simulink model "Fishhook"  (R2018a)
settings: Solver=FixedStepDiscrete  StartTime=0.0  StopTime=1  FixedStep=0.001  RelTol=1e-3  EnableMultiTasking=on
values from neighbouring files (symbols this model uses):
  DLCTest = [0 0 0 0 0 0 0 0 0 0 0 0 ... (12003 elements, 12003x1)]    [DLCTest.mat]
  Ts = 0.001    [ISData.m]    (also in IS_2impulse.m; IS_3impulse.m; IS_4impulse.m; InputShaper.m)
undefined symbols (not defined in the file or in its folder): theta_sw_FH
settings Model: ExtModeTrigDuration=10000  Creator=srivats  LastModifiedBy=srivats
settings SolverCC: PositivePriorityOrder=on
settings RTWCC: SystemTargetFile=quarc_win64.tlc  TemplateMakefile=quarc_default_tmf  Description=QUARC Win64 Target
settings STFCustomTargetCC: TargetPreCompLibLocation=C:\PROGRA~3\QUARC\lib\2018a\win64\release  TargetLangStandard=C99 (ISO)  ConcurrentExecutionCompliant=on  SystemTargetFile=quarc_win64.tlc
settings GRTTargetCC: TargetPreCompLibLocation=C:\PROGRA~3\QUARC\lib\2018a\win64\release  ParMdlRefBuildCompliant=off  CompOptLevelCompliant=off  CombineOutputUpdateFcns=off  MatFileLogging=off  CPPClassGenCompliant=off  GRTInterface=on  UseToolchainInfoCompliant=off  ExtMode=on  ExtModeMexFile=quarc_comm

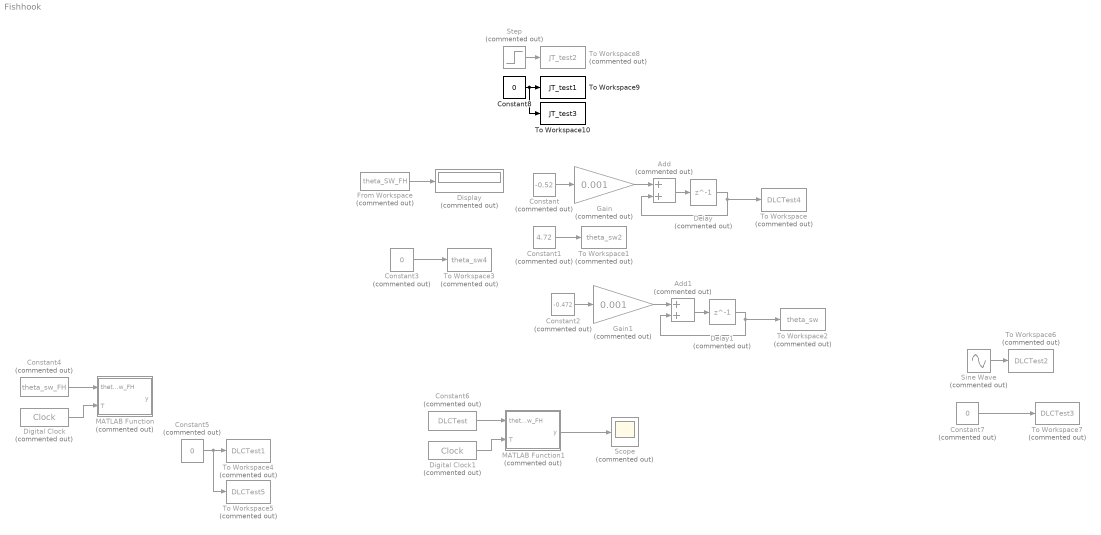
== system Fishhook ==
  Add : Sum  Commented=on
  Add1 : Sum  Commented=on
  Constant : Constant  Commented=on  Value=-0.52
  Constant1 : Constant  Commented=on  Value=4.72
  Constant2 : Constant  Commented=on  Value=-0.472
  Constant3 : Constant  Commented=on  Value=0
  Constant4 : Constant  Commented=on  Value=theta_sw_FH
  Constant5 : Constant  Commented=on  Value=0
  Constant6 : Constant  Commented=on  Value=DLCTest
  Constant7 : Constant  Commented=on  Value=0
  Constant8 : Constant  Value=0
  Delay : Delay  Commented=on  DelayLength=1
  Delay1 : Delay  Commented=on  DelayLength=1  InitialCondition=4.72
  Digital Clock : DigitalClock  Commented=on  SampleTime=0.001
  Digital Clock1 : DigitalClock  Commented=on  SampleTime=0.001
  Display : Display  Commented=on
  From Workspace : FromWorkspace  Commented=on  VariableName=theta_SW_FH  SampleTime=Ts
  Gain : Gain  Commented=on  Gain=0.001
  Gain1 : Gain  Commented=on  Gain=0.001
  MATLAB Function : MATLAB Function  Commented=on  TreatAsAtomicUnit=on
  MATLAB Function1 : MATLAB Function  Commented=on  TreatAsAtomicUnit=on
  Scope : Scope  Commented=on
  Sine Wave : Sin  Commented=on  Amplitude=0.349066  Frequency=2*pi/10  SampleTime=Ts
  Step : Step  Commented=on  After=-3.6  SampleTime=0
  To Workspace : ToWorkspace  Commented=on  VariableName=DLCTest4  SaveFormat=Timeseries  SampleTime=-1
  To Workspace1 : ToWorkspace  Commented=on  VariableName=theta_sw2  SaveFormat=Timeseries  SampleTime=-1
  To Workspace10 : ToWorkspace  VariableName=JT_test3  SaveFormat=Timeseries  SampleTime=-1
  To Workspace2 : ToWorkspace  Commented=on  VariableName=theta_sw  SaveFormat=Timeseries  SampleTime=-1
  To Workspace3 : ToWorkspace  Commented=on  VariableName=theta_sw4  SaveFormat=Timeseries  SampleTime=-1
  To Workspace4 : ToWorkspace  Commented=on  VariableName=DLCTest1  SaveFormat=Timeseries  SampleTime=-1
  To Workspace5 : ToWorkspace  Commented=on  VariableName=DLCTest5  SaveFormat=Timeseries  SampleTime=-1
  To Workspace6 : ToWorkspace  Commented=on  VariableName=DLCTest2  SaveFormat=Timeseries  SampleTime=-1
  To Workspace7 : ToWorkspace  Commented=on  VariableName=DLCTest3  SaveFormat=Timeseries  SampleTime=-1
  To Workspace8 : ToWorkspace  Commented=on  VariableName=JT_test2  SaveFormat=Timeseries  SampleTime=-1
  To Workspace9 : ToWorkspace  VariableName=JT_test1  SaveFormat=Timeseries  SampleTime=-1
  wires:
  Constant/1 -> Gain/1
  Gain/1 -> Add/1
  Add/1 -> Delay/1
  Delay/1 -> To Workspace/1, Add/2
  Constant1/1 -> To Workspace1/1
  Add1/1 -> Delay1/1
  Delay1/1 -> To Workspace2/1, Add1/2
  Gain1/1 -> Add1/1
  Constant2/1 -> Gain1/1
  Constant3/1 -> To Workspace3/1
  From Workspace/1 -> Display/1
  Digital Clock/1 -> MATLAB Function/2(T)
  Constant4/1 -> MATLAB Function/1(theta_sw_FH)
  Constant5/1 -> To Workspace5/1, To Workspace4/1
  Constant6/1 -> MATLAB Function1/1(theta_sw_FH)
  Digital Clock1/1 -> MATLAB Function1/2(T)
  MATLAB Function1/1(y) -> Scope/1
  Sine Wave/1 -> To Workspace6/1
  Constant7/1 -> To Workspace7/1
  Step/1 -> To Workspace8/1
  Constant8/1 -> To Workspace10/1, To Workspace9/1

== matlab function Fishhook/MATLAB Function1 ==
  data: theta_sw_FH input; y output; T input
function y = fcn(theta_sw_FH,T)
    i=(T+0.001)/0.001;
    
y = theta_sw_FH(i);

== matlab function Fishhook/MATLAB Function ==
  data: theta_sw_FH input; y output; T input
function y = fcn(theta_sw_FH,T)
    i=(T+0.001)/0.001;
    
y = theta_sw_FH(i);
